simulink model "LQR"  (R2020a)
settings: Solver=VariableStepAuto  StartTime=0.0  StopTime=20  RelTol=1e-3
values from neighbouring files (symbols this model uses):
  A_23 = -(M^2*L^2*g)/Q    (= -14.1433795261)    [parameter_LQR.m]
  A_43 = M*L*g*(M+2*m+2*inertia/r^2)/Q    (= 410.971610924)    [parameter_LQR.m]
  B_21 = (J_centroid+M*L^2+M*L*r)/(Q*r)    (= 110.773162975)    [parameter_LQR.m]
  B_22 = B_21    (= 110.773162975)    [parameter_LQR.m]
  B_41 = -(M*L/r+M+2*m+2*inertia/r^2)/Q    (= -2383.23139104)    [parameter_LQR.m]
  B_42 = B_41    (= -2383.23139104)    [parameter_LQR.m]
  B_61 = 1/(r*(m*d+inertia*d/r^2+2*J_Y_delata/d))    (= 1721.93672953)    [parameter_LQR.m]
  B_62 = -B_61    (= -1721.93672953)    [parameter_LQR.m]
  K = lqr(A,B,Q,R)    [parameter_LQR.m]
settings Model: Creator=Pascal  LastModifiedBy=Administrator
settings DataIOCC: ReturnWorkspaceOutputs=off
settings DebuggingCC: ArithmeticOperatorsInVariantConditions=warning
settings SFSimCC: CustomCodeUndefinedFunction=UseInterfaceOnly

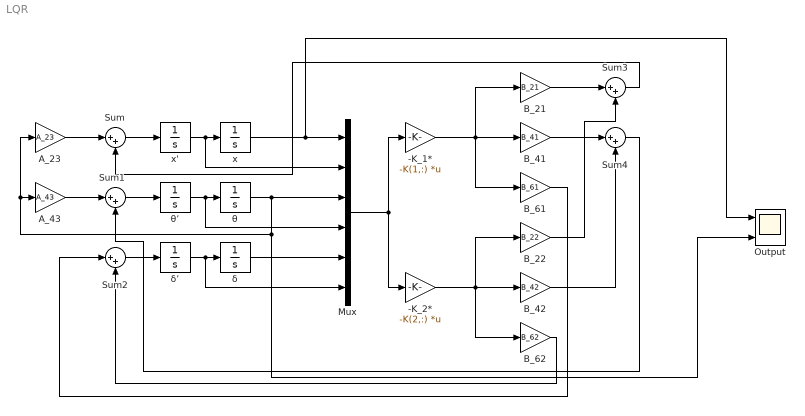
== system LQR ==
  -K_1* : Gain  Gain=-K(1,:)  Multiplication=Matrix(K*u)
  -K_2* : Gain  Gain=-K(2,:)  Multiplication=Matrix(K*u)
  A_23 : Gain  Gain=A_23
  A_43 : Gain  Gain=A_43
  B_21 : Gain  Gain=B_21
  B_22 : Gain  Gain=B_22
  B_41 : Gain  Gain=B_41
  B_42 : Gain  Gain=B_42
  B_61 : Gain  Gain=B_61
  B_62 : Gain  Gain=B_62
  Mux : Mux  Inputs=6
  Output : Scope  NumInputPorts=2
  Sum{,1..4} (5 alike) : Sum  Inputs=|++
  x : Integrator
  x' : Integrator
  δ : Integrator
  δ’ : Integrator
  θ : Integrator  InitialCondition=0.7
  θ’ : Integrator  InitialCondition=0.2
  wires:
  x'/1 -> Mux/2, x/1
  -K_2*/1 -> B_22/1, B_42/1, B_62/1
  θ/1 -> A_23/1, A_43/1, Output/2, Mux/3
  Sum4/1 -> Sum1/2
  Sum1/1 -> θ’/1
  B_41/1 -> Sum4/1
  Sum3/1 -> Sum/2
  Sum/1 -> x'/1
  Mux/1 -> -K_2*/1, -K_1*/1
  B_22/1 -> Sum3/2
  Sum2/1 -> δ’/1
  B_62/1 -> Sum2/2
  A_23/1 -> Sum/1
  δ’/1 -> Mux/6, δ/1
  -K_1*/1 -> B_21/1, B_41/1, B_61/1
  B_61/1 -> Sum2/1
  A_43/1 -> Sum1/1
  δ/1 -> Mux/5
  B_21/1 -> Sum3/1
  x/1 -> Output/1, Mux/1
  θ’/1 -> Mux/4, θ/1
  B_42/1 -> Sum4/2
